simulink model "Bus_test1"  (R2024a)
settings: Solver=FixedStepAuto  StartTime=0.0  StopTime=10  FixedStep=0.01  RelTol=1e-3
libraries: svdutilitieslib x1, dspnetwork x1
settings Model: PacingRate=0.100000  Creator=azmol  LastModifiedBy=azmol
settings SolverCC: AutoInsertRateTranBlk=on  InsertRTBMode=Never (minimum delay)

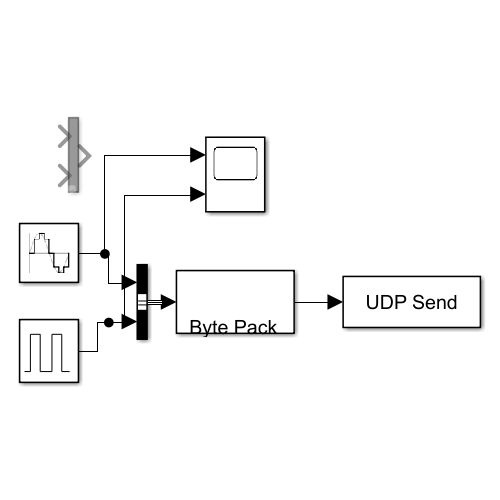
[thumbnail: Simulink's stored preview of the top-level diagram]
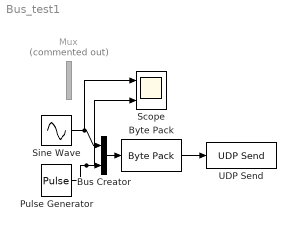
== system Bus_test1 ==
  Bus Creator : BusCreator  Inputs=2
  Byte Pack : svdutilitieslib/Byte Pack  maskPackedDataType=uint8  datatypes={'double'}  byteAlign=1  blockPlatform=tic2000
      settings: LibrarySourceBlock=c2000lib/Target Communication/Byte Pack
  Mux : Mux  Commented=on  Inputs=2
  Pulse Generator : DiscretePulseGenerator  PulseType=Time based  Period=3.5  PulseWidth=50
  Scope : Scope  NumInputPorts=2
  Sine Wave : Sin
  UDP Send : dspnetwork/UDP Send  remoteURL='127.0.0.1'  remotePort=25001  localURL='0.0.0.0'  localPortSource=Automatically determine  localPort=-1  sendBufferSize=8192  sampletime=-1  blockPlatform=[]  separateLengthPort=0
      settings: LibrarySourceBlock=dspsnks4/UDP Send
  wires:
  Sine Wave/1 -> Scope/1, Bus Creator/1
  Pulse Generator/1 -> Scope/2, Bus Creator/2
  Bus Creator/1 -> Byte Pack/1
  Byte Pack/1 -> UDP Send/1
